simulink library "send"  (R2024a)
settings: Solver=VariableStepAuto  StartTime=0.0  StopTime=10.0  RelTol=1e-3
settings Model: Creator=eikel  LastModifiedBy=adriaeik

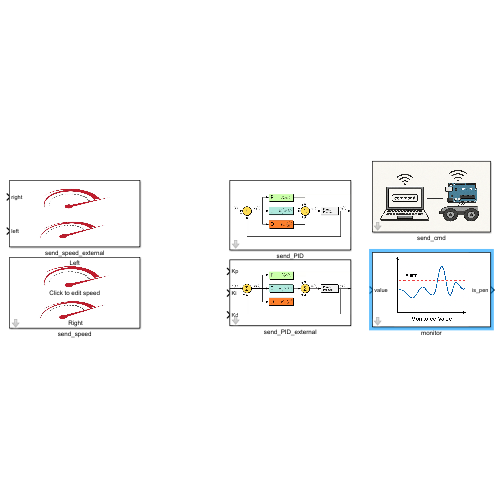
[thumbnail: Simulink's stored preview of the top-level diagram]
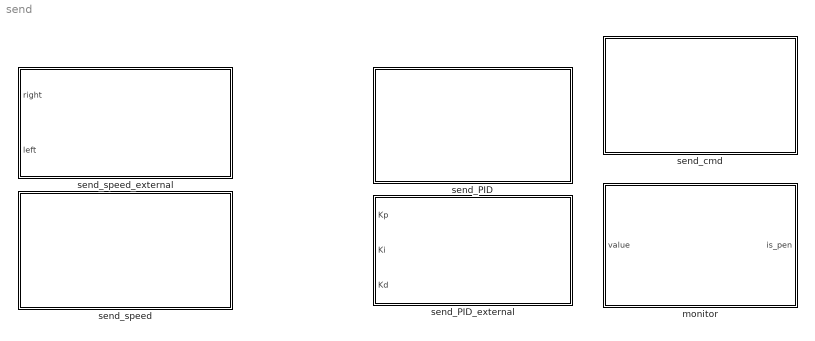
== system send ==
  monitor : Subsystem
      mask Display: image('avvik.png', [0,0,0,0,100,100]);
  send_PID : Subsystem  mask{kp=0, ki=0, kd=0}
      mask prompts: kp "Kp (Proportional term)"; ki "Ki (Integral term)"; kd "Kd (Derivative term)"
      mask Display: image('PID.png', [0,0,0,0,100,80]);
  send_PID_external : Subsystem
      mask Display: image('PID.png', [0,0,0,0,100,80]);
  send_cmd : Subsystem  mask{cmd=Start}
      mask prompts: cmd "Command"
      mask TypeOptions cmd: Start | Stop | Manual | PID-mode | Calibrate
      mask Display: image('command.png');
  send_speed : Subsystem  mask{left=0, right=0}
      mask Display:
      | image('speed.jpg');
      | disp(['Left\n\n\n\n' ...
      |     'Click to edit speed\n\n\n\n ' ...
      |     'Right']);
  send_speed_external : Subsystem
      mask Display: image('speed.jpg');

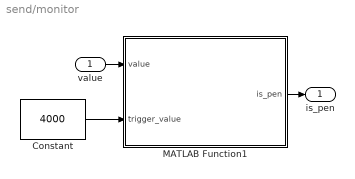
== system send/monitor ==
  value : Inport
  Constant : Constant  Value=4000
  MATLAB Function1 : MATLAB Function  TreatAsAtomicUnit=on
  is_pen : Outport
  wires:
  Constant/1 -> MATLAB Function1/2(trigger_value)
  value/1 -> MATLAB Function1/1(value)
  MATLAB Function1/1(is_pen) -> is_pen/1

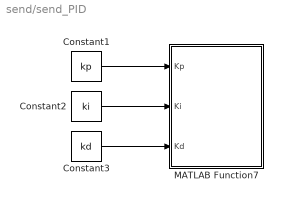
== system send/send_PID ==
  Constant1 : Constant  Value=kp
  Constant2 : Constant  Value=ki
  Constant3 : Constant  Value=kd
  MATLAB Function7 : MATLAB Function  TreatAsAtomicUnit=on
  wires:
  Constant1/1 -> MATLAB Function7/1(Kp)
  Constant2/1 -> MATLAB Function7/2(Ki)
  Constant3/1 -> MATLAB Function7/3(Kd)

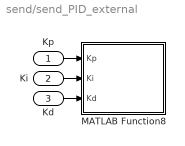
== system send/send_PID_external ==
  Kp : Inport
  Ki : Inport  Port=2
  Kd : Inport  Port=3
  MATLAB Function8 : MATLAB Function  TreatAsAtomicUnit=on
  wires:
  Kp/1 -> MATLAB Function8/1(Kp)
  Kd/1 -> MATLAB Function8/3(Kd)
  Ki/1 -> MATLAB Function8/2(Ki)

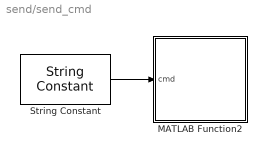
== system send/send_cmd ==
  MATLAB Function2 : MATLAB Function  TreatAsAtomicUnit=on
  String Constant : StringConstant  String=cmd
  wires:
  String Constant/1 -> MATLAB Function2/1(cmd)

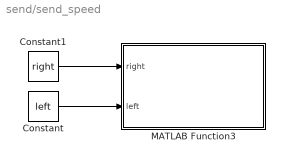
== system send/send_speed ==
  Constant : Constant  Value=left
  Constant1 : Constant  Value=right
  MATLAB Function3 : MATLAB Function  TreatAsAtomicUnit=on
  wires:
  Constant/1 -> MATLAB Function3/2(left)
  Constant1/1 -> MATLAB Function3/1(right)

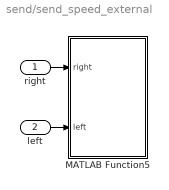
== system send/send_speed_external ==
  right : Inport
  left : Inport  Port=2
  MATLAB Function5 : MATLAB Function  TreatAsAtomicUnit=on
  wires:
  left/1 -> MATLAB Function5/2(left)
  right/1 -> MATLAB Function5/1(right)

== matlab function send/send_cmd/MATLAB Function2 ==
  data: cmd input
function publish_cmd(cmd)
    coder.extrinsic('send_cmd');

    persistent last_cmd
    if isempty(last_cmd)
        last_cmd = blanks(20);  % 1x20 char-array
    end

    % Konverter input til char
    cmd_char = char(cmd);
    L = length(cmd_char);

    % Sørg for at cmd_padded er ALLTID 1x20
    cmd_padded = blanks(20);      % Alloker fast lengde
    N = min(L, 20);               % maks 20 teikn
    cmd_padded(1:N) = cmd_char(1:N);  % kopier teikna

    % Samanlikn og send berre ved endring
    if ~strcmp(cmd_padded, last_cmd)
        send_cmd(strtrim(cmd_padded));  % send utan whitespace
        last_cmd = cmd_padded;          % lagre nytt for samanlikning
        if last_cmd ~= blanks(20)
            last_cmd = blanks(20);
        end
    end
end

== matlab function send/send_speed/MATLAB Function3 ==
  data: right input; left input
function publish_speed(right, left)
    coder.extrinsic('send_speed');  % kallar på ekstern MATLAB-funksjon

    persistent last_right last_left

    if isempty(last_right)
        last_right = NaN;
        last_left  = NaN;
    end

    if right ~= last_right || left ~= last_left
        send_speed(left, right); % berre send om verdiar har endra seg
        last_right = right;
        last_left  = left;
    end
end

== matlab function send/send_speed_external/MATLAB Function5 ==
  data: right input; left input
function publish_speed(right, left)
    coder.extrinsic('send_speed');  % merk: dette peikar på .m-fila di
    send_speed(left, right)
end

== matlab function send/send_PID/MATLAB Function7 ==
  data: Kp input; Ki input; Kd input
function publish_PID(Kp, Ki, Kd)
    coder.extrinsic('send_PID');  

    persistent last_Kp last_Ki last_Kd

    if isempty(last_Kp)
        last_Kp = NaN; % sørg for første utsending
        last_Ki = NaN;
        last_Kd = NaN;
    end

    % Sjekk om noko har endra seg
    if Kp ~= last_Kp || Ki ~= last_Ki || Kd ~= last_Kd
        send_PID(Kp, Ki, Kd); % send berre om noko endra seg
        last_Kp = Kp;
        last_Ki = Ki;
        last_Kd = Kd;
    end
end

== matlab function send/send_PID_external/MATLAB Function8 ==
  data: Kp input; Ki input; Kd input
function publish_PID(Kp, Ki, Kd)
    coder.extrinsic('send_PID');  

    persistent last_Kp last_Ki last_Kd

    if isempty(last_Kp)
        last_Kp = NaN; % sørg for første utsending
        last_Ki = NaN;
        last_Kd = NaN;
    end

    % Sjekk om noko har endra seg
    if Kp ~= last_Kp || Ki ~= last_Ki || Kd ~= last_Kd
        send_PID(Kp, Ki, Kd); % send berre om noko endra seg
        last_Kp = Kp;
        last_Ki = Ki;
        last_Kd = Kd;
    end
end

== matlab function send/monitor/MATLAB Function1 ==
  settings: updateMethod=DISCRETE
  data: value input; is_pen output; trigger_value input
function is_pen = publish_penalty(value, trigger_value)
    coder.extrinsic('send_penalty');

    persistent last_cmd
    if isempty(last_cmd)
        last_cmd = 0;  % tom int
    end

    
    if value > trigger_value
        is_pen = true;
        cmd = 1;
    else
        is_pen = false;
        cmd = 0;
    end

    if cmd ~= last_cmd
        send_penalty(cmd);
        last_cmd = cmd;
    end
end
